simulink model "Separador"  (R2017b)
settings: Solver=VariableStepAuto  StartTime=0.0  StopTime=3000  RelTol=1e-3
values from neighbouring files (symbols this model uses):
  D1 = x(3)    [pid_separador.m]
  D2 = x(6)    [pid_separador.m]
  I1 = x(2)    [pid_separador.m]
  I2 = x(5)    [pid_separador.m]
  k1 = sym2poly(Ff_lo * Flo_xl)/a    [pid_separador.m]
  k2 = sym2poly(Ff_li)/a    [pid_separador.m]
  k3 = sym2poly(Ff_lo * Flo_p)/a    [pid_separador.m]
  k4 = sym2poly(Fg_li) /den    [pid_separador.m]
  k5 = sym2poly(Fg_gi)/den    [pid_separador.m]
  k6 = sym2poly(Fg_lo* Flo_xl) /den    [pid_separador.m]
  k7 = sym2poly((Fg_lo* Flo_hl)+(Fg_vl*Fvl_hl))/den    [pid_separador.m]
  k8 = sym2poly(Fg_go* Fgo_xg) /den    [pid_separador.m]
  k9 = sym2poly(Fg_go* Fgo_t) /den    [pid_separador.m]
  P1 = x(1)    [pid_separador.m]
  P2 = x(4)    [pid_separador.m]
  tau1 = 1/a    [pid_separador.m]
  tau2 = 1/a    [pid_separador.m]
  tau3 = tau1    [pid_separador.m]
  tau4 = 1 /den    [pid_separador.m]
  tau5 = tau4    [pid_separador.m]
  tau6 = tau4    [pid_separador.m]
  tau7 = tau4    [pid_separador.m]
  tau8 = tau4    [pid_separador.m]
  tau9 = tau4    [pid_separador.m]
libraries: simulink x2
settings Model: Creator=Rafael Azambuja  LastModifiedBy=Rafael Azambuja

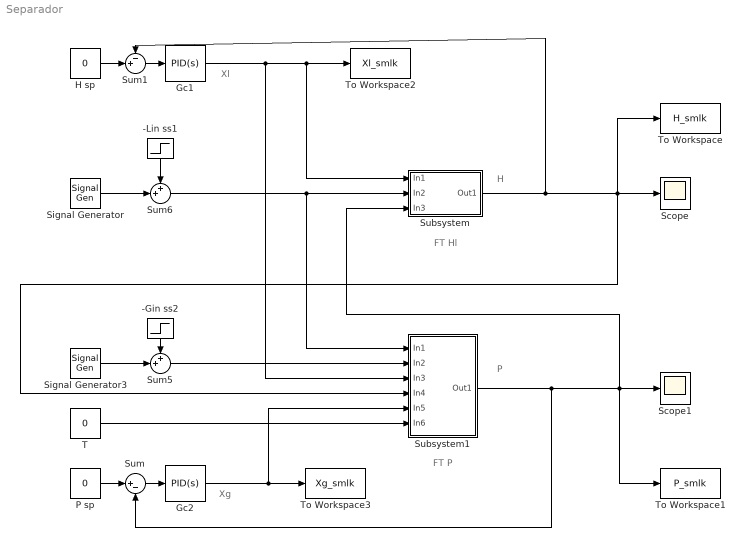
== system Separador ==
  note: Xg
  note: Xl
  note: FT P
  note: P
  note: FT Hl
  note: H
  -Gin ss2 : Step  Time=0  After=0  SampleTime=0
  -Lin ss1 : Step  Time=0  After=0  SampleTime=0
  Gc1 : simulink/Continuous/PID Controller  Controller=PID  TimeDomain=Continuous-time  SampleTime=-1  IntegratorMethod=Forward Euler  FilterMethod=Forward Euler  Form=Parallel  UseFilter=on  ControllerParametersSource=internal  P=P1  I=I1  D=D1  N=100  InitialConditionSource=internal  InitialConditionForIntegrator=0  InitialConditionForFilter=0  ExternalReset=none  LimitOutput=off  UpperSaturationLimit=inf  LowerSaturationLimit=-inf  LinearizeAsGain=off  AntiWindupMode=none  Kb=1  TrackingMode=off  Kt=1  PParamMin=[]  PParamMax=[]  IParamMin=[]  IParamMax=[]  DParamMin=[]  DParamMax=[]  NParamMin=[]  NParamMax=[]  KbParamMin=[]  KbParamMax=[]  KtParamMin=[]  KtParamMax=[]  POutMin=[]  POutMax=[]  IOutMin=[]  IOutMax=[]  DOutMin=[]  DOutMax=[]  NOutMin=[]  NOutMax=[]  KbOutMin=[]  KbOutMax=[]  KtOutMin=[]  KtOutMax=[]  IntegratorOutMin=[]  IntegratorOutMax=[]  FilterOutMin=[]  FilterOutMax=[]  SumOutMin=[]  SumOutMax=[]  SumI1OutMin=[]  SumI1OutMax=[]  SumI2OutMin=[]  SumI2OutMax=[]  SumI3OutMin=[]  SumI3OutMax=[]  SumDOutMin=[]  SumDOutMax=[]  SaturationOutMin=[]  SaturationOutMax=[]  IntegratorContinuousStateAttributes=''  IntegratorStateMustResolveToSignalObject=off  IntegratorRTWStateStorageClass=Auto  FilterContinuousStateAttributes=''  FilterStateMustResolveToSignalObject=off  FilterRTWStateStorageClass=Auto  DifferentiatorICPrevScaledInput=0  DifferentiatorOutMin=[]  DifferentiatorOutMax=[]  InitialConditionSetting=State (most efficient)  FilterDiffOutCoefMin=[]  FilterDiffOutCoefMax=[]  SumDenOutMin=[]  SumDenOutMax=[]  SumNumOutMin=[]  SumNumOutMax=[]  ReciprocalOutMin=[]  ReciprocalOutMax=[]  DivideOutMin=[]  DivideOutMax=[]  TunerSelectOption=Transfer Function Based (PID Tuner App)
  Gc2 : simulink/Continuous/PID Controller  Controller=PID  TimeDomain=Continuous-time  SampleTime=-1  IntegratorMethod=Forward Euler  FilterMethod=Forward Euler  Form=Parallel  UseFilter=on  ControllerParametersSource=internal  P=P2  I=I2  D=D2  N=100  InitialConditionSource=internal  InitialConditionForIntegrator=0  InitialConditionForFilter=0  ExternalReset=none  LimitOutput=off  UpperSaturationLimit=inf  LowerSaturationLimit=-inf  LinearizeAsGain=off  AntiWindupMode=none  Kb=1  TrackingMode=off  Kt=1  PParamMin=[]  PParamMax=[]  IParamMin=[]  IParamMax=[]  DParamMin=[]  DParamMax=[]  NParamMin=[]  NParamMax=[]  KbParamMin=[]  KbParamMax=[]  KtParamMin=[]  KtParamMax=[]  POutMin=[]  POutMax=[]  IOutMin=[]  IOutMax=[]  DOutMin=[]  DOutMax=[]  NOutMin=[]  NOutMax=[]  KbOutMin=[]  KbOutMax=[]  KtOutMin=[]  KtOutMax=[]  IntegratorOutMin=[]  IntegratorOutMax=[]  FilterOutMin=[]  FilterOutMax=[]  SumOutMin=[]  SumOutMax=[]  SumI1OutMin=[]  SumI1OutMax=[]  SumI2OutMin=[]  SumI2OutMax=[]  SumI3OutMin=[]  SumI3OutMax=[]  SumDOutMin=[]  SumDOutMax=[]  SaturationOutMin=[]  SaturationOutMax=[]  IntegratorContinuousStateAttributes=''  IntegratorStateMustResolveToSignalObject=off  IntegratorRTWStateStorageClass=Auto  FilterContinuousStateAttributes=''  FilterStateMustResolveToSignalObject=off  FilterRTWStateStorageClass=Auto  DifferentiatorICPrevScaledInput=0  DifferentiatorOutMin=[]  DifferentiatorOutMax=[]  InitialConditionSetting=State (most efficient)  FilterDiffOutCoefMin=[]  FilterDiffOutCoefMax=[]  SumDenOutMin=[]  SumDenOutMax=[]  SumNumOutMin=[]  SumNumOutMax=[]  ReciprocalOutMin=[]  ReciprocalOutMax=[]  DivideOutMin=[]  DivideOutMax=[]  TunerSelectOption=Transfer Function Based (PID Tuner App)
  H sp : Constant  Value=0
  P sp : Constant  Value=0
  Scope : Scope
  Scope1 : Scope
  Signal Generator : SignalGenerator  Amplitude=0.05  Frequency=1/1320
  Signal Generator3 : SignalGenerator  Amplitude=0.0928  Frequency=1/1320
  Subsystem : Subsystem
  Subsystem1 : Subsystem
  Sum : Sum  Inputs=|+-
  Sum1 : Sum  Inputs=-+|
  Sum5 : Sum  Inputs=++|
  Sum6 : Sum  Inputs=++|
  T : Constant  Value=0
  To Workspace : ToWorkspace  VariableName=H_smlk  SaveFormat=Timeseries  SampleTime=1
  To Workspace1 : ToWorkspace  VariableName=P_smlk  SaveFormat=Timeseries  SampleTime=1
  To Workspace2 : ToWorkspace  VariableName=Xl_smlk  SaveFormat=Timeseries  SampleTime=1
  To Workspace3 : ToWorkspace  VariableName=Xg_smlk  SaveFormat=Timeseries  SampleTime=1
  wires:
  Signal Generator3/1 -> Sum5/2
  -Lin ss1/1 -> Sum6/1
  Subsystem1/1(Out1) -> Sum/2, To Workspace1/1, Scope1/1, Subsystem/3(In3)
  Subsystem/1(Out1) -> Sum1/1, To Workspace/1, Scope/1, Subsystem1/4(In4)
  Sum5/1 -> Subsystem1/2(In2)
  Gc1/1 -> Subsystem1/3(In3), Subsystem/1(In1), To Workspace2/1
  Sum6/1 -> Subsystem1/1(In1), Subsystem/2(In2)
  Signal Generator/1 -> Sum6/2
  T/1 -> Subsystem1/6(In6)
  -Gin ss2/1 -> Sum5/1
  Gc2/1 -> To Workspace3/1, Subsystem1/5(In5)
  Sum1/1 -> Gc1/1
  H sp/1 -> Sum1/2
  Sum/1 -> Gc2/1
  P sp/1 -> Sum/1

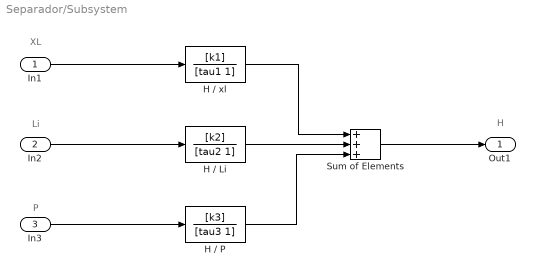
== system Separador/Subsystem ==
  note: H
  note: P
  note: Li
  note: XL
  In1 : Inport
  In2 : Inport  Port=2
  In3 : Inport  Port=3
  H / Li : TransferFcn  Numerator=[k2]  Denominator=[tau2 1]
  H / P : TransferFcn  Numerator=[k3]  Denominator=[tau3 1]
  H / xl : TransferFcn  Numerator=[k1]  Denominator=[tau1 1]
  Sum of Elements : Sum  Inputs=+++
  Out1 : Outport
  wires:
  In1/1 -> H / xl/1
  In2/1 -> H / Li/1
  In3/1 -> H / P/1
  H / xl/1 -> Sum of Elements/1
  H / Li/1 -> Sum of Elements/2
  H / P/1 -> Sum of Elements/3
  Sum of Elements/1 -> Out1/1

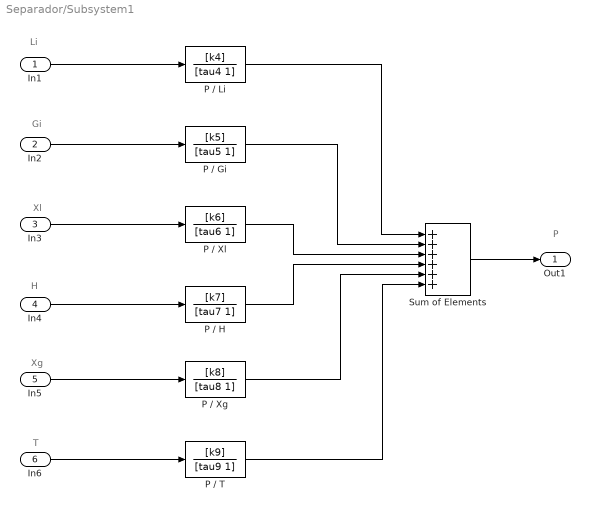
== system Separador/Subsystem1 ==
  note: T
  note: Xg
  note: H
  note: P
  note: Xl
  note: Gi
  note: Li
  In1 : Inport
  In2 : Inport  Port=2
  In3 : Inport  Port=3
  In4 : Inport  Port=4
  In5 : Inport  Port=5
  In6 : Inport  Port=6
  P / Gi : TransferFcn  Numerator=[k5]  Denominator=[tau5 1]
  P / H : TransferFcn  Numerator=[k7]  Denominator=[tau7 1]
  P / Li : TransferFcn  Numerator=[k4]  Denominator=[tau4 1]
  P / T : TransferFcn  Numerator=[k9]  Denominator=[tau9 1]
  P / Xg : TransferFcn  Numerator=[k8]  Denominator=[tau8 1]
  P / Xl : TransferFcn  Numerator=[k6]  Denominator=[tau6 1]
  Sum of Elements : Sum  Inputs=++++++
  Out1 : Outport
  wires:
  In1/1 -> P / Li/1
  In2/1 -> P / Gi/1
  In3/1 -> P / Xl/1
  Sum of Elements/1 -> Out1/1
  In4/1 -> P / H/1
  In5/1 -> P / Xg/1
  In6/1 -> P / T/1
  P / T/1 -> Sum of Elements/6
  P / Xg/1 -> Sum of Elements/5
  P / H/1 -> Sum of Elements/4
  P / Xl/1 -> Sum of Elements/3
  P / Gi/1 -> Sum of Elements/2
  P / Li/1 -> Sum of Elements/1
